simulink model "PathPlanning"  (R2025a)
settings: Solver=FixedStepAuto  StartTime=0.0  StopTime=10  FixedStep=1  RelTol=1e-3  EnableMultiTasking=on
undefined symbols (not defined in the file): costMap, finalPose, geometry, initialPose, metric, samplingBoxCenterPose, samplingBoxDimension, verticesStaticObstacles
libraries: MPSV x3
settings Model: Creator=damerius  LastModifiedBy=damerius
settings SolverCC: ConcurrentTasks=on  AlgebraicLoopSolver=TrustRegion  PositivePriorityOrder=on
settings DataIOCC: SaveOutput=off  SignalLogging=off  DSMLogging=off  SaveTime=off  ReturnWorkspaceOutputs=off
settings OptimizationCC: DefaultParameterBehavior=Inlined  ReuseModelBlockBuffer=off  ZeroExternalMemoryAtStartup=off  ZeroInternalMemoryAtStartup=off  SimCompilerOptimization=on
settings DebuggingCC: UnconnectedInputMsg=warning  UnconnectedOutputMsg=warning  UnconnectedLineMsg=warning
settings HardwareCC: ProdBitPerLong=64.0  ProdHWDeviceType=Intel->x86-64 (Linux 64)
settings ModelReferenceCC: EnableRefExpFcnMdlSchedulingChecks=on
settings SFSimCC: SimParseCustomCode=off  SimGenImportedTypeDefs=on  SimTargetLang=C++  SimDLTargetLibrary=mkl-dnn
settings RTWCC: GenCodeOnly=on  PackageGeneratedCodeAndArtifacts=on  PackageName=PackNGo  RTWVerbose=off  BuildConfiguration=Faster Runs  TargetLang=C++  GPUComputeCapability=3.5  DLArmComputeVersion=19.05
settings CodeAppCC: ForceParamTrailComments=on  MaxIdLength=95.0  MATLABSourceComments=on  UseSimReservedNames=on
settings GRTTargetCC: TargetLangStandard=C++11 (ISO)  GenerateFullHeader=off  MatFileLogging=off  CodeInterfacePackaging=C++ class  SubcomponentCodeInterfacePackaging=C++ class

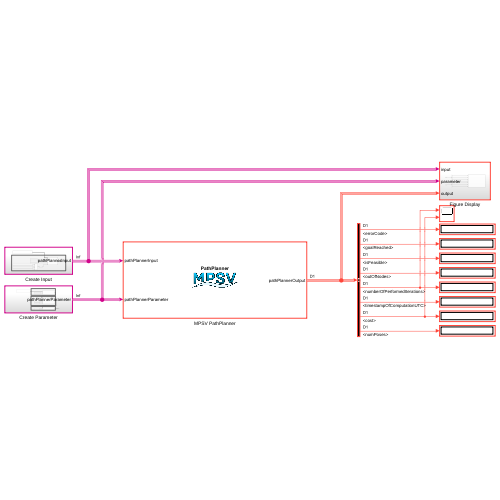
[thumbnail: Simulink's stored preview of the top-level diagram]
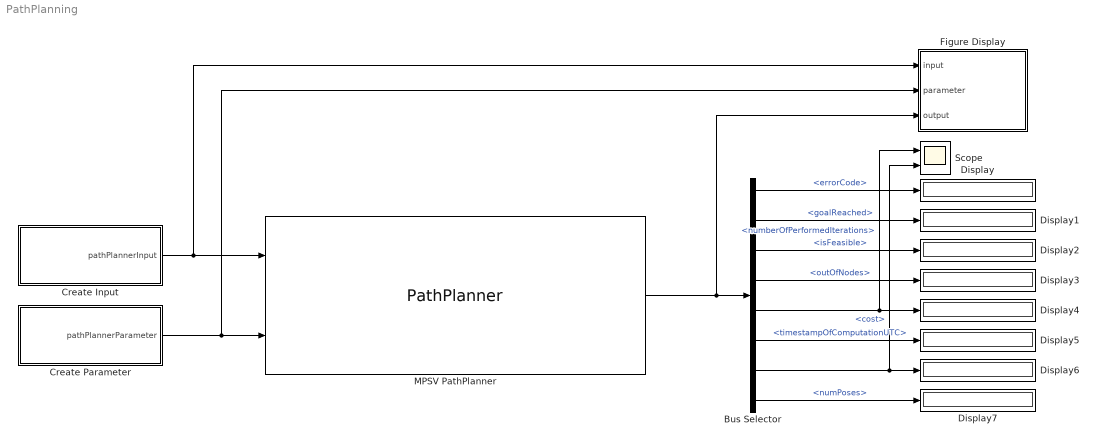
== system PathPlanning ==
  Bus Selector : BusSelector  OutputSignals=errorCode,goalReached,isFeasible,outOfNodes,numberOfPerformedIterations,timestampOfComputationUTC,cost,numPoses
  Create Input : Subsystem
  Create Parameter : Subsystem
  Display{,1..7} (8 alike) : Display
  Figure Display : Subsystem
  MPSV PathPlanner : MPSV/PathPlanner  maxNumNodes=1000  maxNumSamples=1000000
      settings: SourceProductName=MPSV - Motion Planner for Surface Vehicles
  Scope : Scope  NumInputPorts=2
      settings: ActiveDisplayYMinimum=19472  ActiveDisplayYMaximum=20852
  wires:
  MPSV PathPlanner/1 -> Figure Display/3(output), Bus Selector/1
  Bus Selector/8 -> Display7/1  "<numPoses>"
  Bus Selector/7 -> Scope/2, Display6/1  "<cost>"
  Bus Selector/6 -> Display5/1  "<timestampOfComputationUTC>"
  Bus Selector/5 -> Scope/1, Display4/1  "<numberOfPerformedIterations>"
  Create Input/1(pathPlannerInput) -> Figure Display/1(input), MPSV PathPlanner/1
  Create Parameter/1(pathPlannerParameter) -> Figure Display/2(parameter), MPSV PathPlanner/2
  Bus Selector/1 -> Display/1  "<errorCode>"
  Bus Selector/2 -> Display1/1  "<goalReached>"
  Bus Selector/3 -> Display2/1  "<isFeasible>"
  Bus Selector/4 -> Display3/1  "<outOfNodes>"

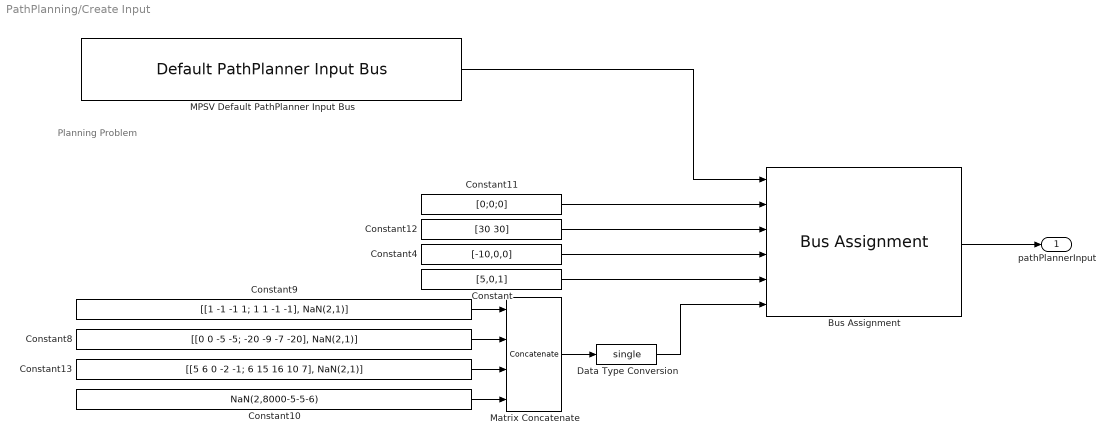
== system PathPlanning/Create Input ==
  note: Planning Problem
  Bus Assignment : BusAssignment  AssignedSignals=samplingBoxCenterPose,samplingBoxDimension,initialPose,finalPose,verticesStaticObstacles
  Constant : Constant  Value=[5,0,1]
  Constant10 : Constant  Value=NaN(2,8000-5-5-6)
  Constant11 : Constant  Value=[0;0;0]
  Constant12 : Constant  Value=[30 30]
  Constant13 : Constant  Value=[[5 6 0 -2 -1; 6 15 16 10 7], NaN(2,1)]
  Constant4 : Constant  Value=[-10,0,0]
  Constant8 : Constant  Value=[[0 0 -5 -5; -20 -9 -7 -20], NaN(2,1)]
  Constant9 : Constant  Value=[[1 -1 -1 1; 1 1 -1 -1], NaN(2,1)]
  Data Type Conversion : DataTypeConversion  OutDataTypeStr=single  SaturateOnIntegerOverflow=off  RndMeth=Floor
  MPSV Default PathPlanner Input Bus : MPSV/Default PathPlanner Input Bus
      settings: SourceProductName=MPSV - Motion Planner for Surface Vehicles
  Matrix Concatenate : Concatenate  NumInputs=4  Mode=Multidimensional array  ConcatenateDimension=2
  pathPlannerInput : Outport
  wires:
  Constant11/1 -> Bus Assignment/2
  Constant/1 -> Bus Assignment/5
  Constant4/1 -> Bus Assignment/4
  MPSV Default PathPlanner Input Bus/1 -> Bus Assignment/1
  Constant12/1 -> Bus Assignment/3
  Bus Assignment/1 -> pathPlannerInput/1
  Constant8/1 -> Matrix Concatenate/2
  Constant13/1 -> Matrix Concatenate/3
  Constant10/1 -> Matrix Concatenate/4
  Constant9/1 -> Matrix Concatenate/1
  Matrix Concatenate/1 -> Data Type Conversion/1
  Data Type Conversion/1 -> Bus Assignment/6

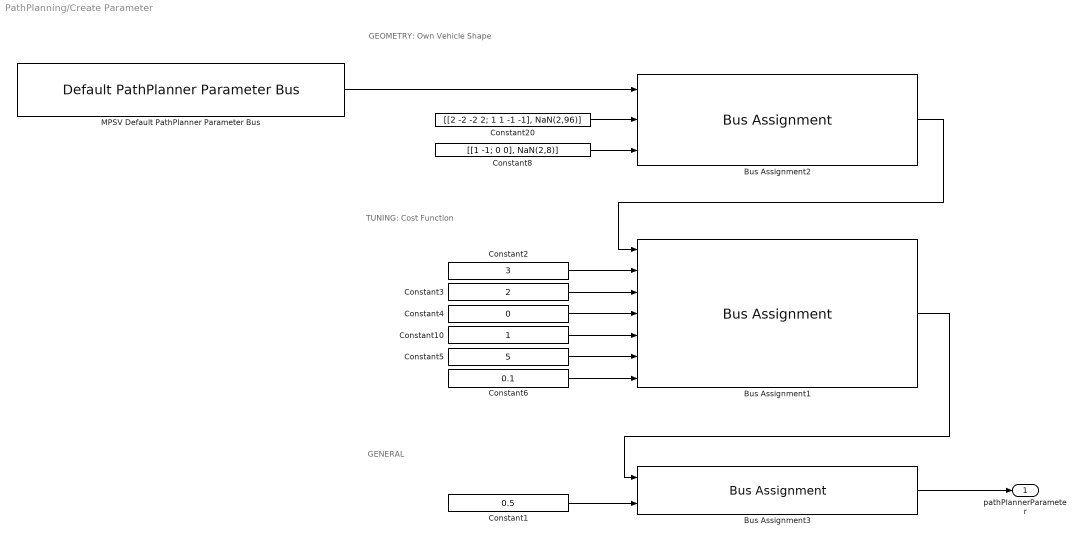
== system PathPlanning/Create Parameter ==
  note: GEOMETRY: Own Vehicle Shape
  note: TUNING: Cost Function
  note: GENERAL
  Bus Assignment1 : BusAssignment  AssignedSignals=metric.weightPsi,metric.weightSway,metric.weightReverseScale,metric.weightReverseDecay,costMap.distanceScale,costMap.distanceDecay
  Bus Assignment2 : BusAssignment  AssignedSignals=geometry.verticesVehicleShape,geometry.skeletalPoints
  Bus Assignment3 : BusAssignment  AssignedSignals=pathPlanner.maxComputationTime
  Constant1 : Constant  Value=0.5
  Constant10 : Constant
  Constant2 : Constant  Value=3
  Constant20 : Constant  Value=[[2 -2 -2 2; 1 1 -1 -1], NaN(2,96)]  OutDataTypeStr=single
  Constant3 : Constant  Value=2
  Constant4 : Constant  Value=0
  Constant5 : Constant  Value=5
  Constant6 : Constant  Value=0.1
  Constant8 : Constant  Value=[[1 -1; 0 0], NaN(2,8)]  OutDataTypeStr=single
  MPSV Default PathPlanner Parameter Bus : MPSV/Default PathPlanner Parameter Bus
      settings: SourceProductName=MPSV - Motion Planner for Surface Vehicles
  pathPlannerParameter : Outport
  wires:
  Constant8/1 -> Bus Assignment2/3
  Constant5/1 -> Bus Assignment1/6
  MPSV Default PathPlanner Parameter Bus/1 -> Bus Assignment2/1
  Constant1/1 -> Bus Assignment3/2
  Constant2/1 -> Bus Assignment1/2
  Bus Assignment1/1 -> Bus Assignment3/1
  Bus Assignment2/1 -> Bus Assignment1/1
  Constant6/1 -> Bus Assignment1/7
  Constant3/1 -> Bus Assignment1/3
  Bus Assignment3/1 -> pathPlannerParameter/1
  Constant4/1 -> Bus Assignment1/4
  Constant10/1 -> Bus Assignment1/5
  Constant20/1 -> Bus Assignment2/2

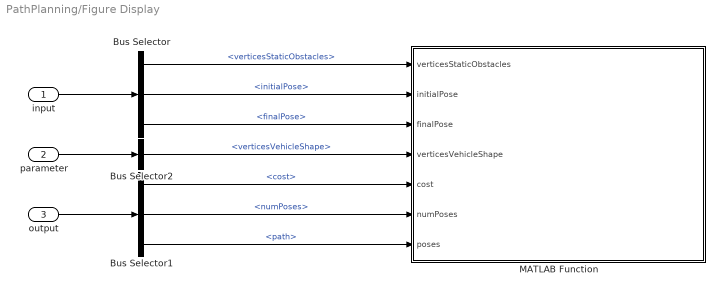
== system PathPlanning/Figure Display ==
  input : Inport
  parameter : Inport  Port=2
  output : Inport  Port=3
  Bus Selector : BusSelector  OutputSignals=verticesStaticObstacles,initialPose,finalPose
  Bus Selector1 : BusSelector  OutputSignals=cost,numPoses,path
  Bus Selector2 : BusSelector  OutputSignals=geometry.verticesVehicleShape
  MATLAB Function : MATLAB Function  TreatAsAtomicUnit=on
  wires:
  parameter/1 -> Bus Selector2/1
  input/1 -> Bus Selector/1
  Bus Selector/1 -> MATLAB Function/1(verticesStaticObstacles)  "<verticesStaticObstacles>"
  Bus Selector/2 -> MATLAB Function/2(initialPose)  "<initialPose>"
  Bus Selector/3 -> MATLAB Function/3(finalPose)  "<finalPose>"
  output/1 -> Bus Selector1/1
  Bus Selector1/1 -> MATLAB Function/5(cost)  "<cost>"
  Bus Selector1/2 -> MATLAB Function/6(numPoses)  "<numPoses>"
  Bus Selector1/3 -> MATLAB Function/7(poses)  "<path>"
  Bus Selector2/1 -> MATLAB Function/4(verticesVehicleShape)  "<verticesVehicleShape>"

== matlab function PathPlanning/Figure Display/MATLAB Function ==
  data: verticesStaticObstacles input; initialPose input; finalPose input; verticesVehicleShape input; cost input; numPoses input; poses input
function FigureDisplay(verticesStaticObstacles, initialPose, finalPose, verticesVehicleShape, cost, numPoses, poses)
    persistent f;
    if(isempty(f))
        f = figure(42);
    end

    clf;
    hold on;
    PlotPath(numPoses, poses, verticesVehicleShape, [0 0.3 0.5]);
    PlotVehicleShape(initialPose, verticesVehicleShape, [0.9 0 0]);
    PlotVehicleShape(finalPose, verticesVehicleShape, [0 0.7 0]);
    PlotObstacles(verticesStaticObstacles);
    view(90,-90);
    axis equal;
    box on;
    grid on;
    xlabel('x in m');
    ylabel('y in m');
    title(sprintf('cost: %f',cost));
    drawnow();
end

function PlotPath(numPoses, poses, verticesVehicleShape, color)
    x = poses(1,1:numPoses);
    y = poses(2,1:numPoses);
    plot(x,y,'LineWidth',2,'Color',color);
    for i = uint32(1):uint32(numPoses)
        PlotVehicleShape(poses(:,i), verticesVehicleShape, color);
    end
end

function PlotVehicleShape(pose, verticesVehicleShape, color)
    c = cos(pose(3));
    s = sin(pose(3));
    R = [c -s; s c];

    N = int32(size(verticesVehicleShape,2));
    i0 = int32(-1);

    for i = int32(1):N
        finiteVertex = isfinite(verticesVehicleShape(1,i)) && isfinite(verticesVehicleShape(2,i));
        if((i0 < 1) && finiteVertex)
            i0 = i;
        elseif((i0 > 0) && (~finiteVertex || (i == N)))
            i = i + int32((i == N) && finiteVertex);
            vertices = R * verticesVehicleShape(:,i0:(i-1)) + [pose(1); pose(2)];
            PlotPolygon(vertices, color);
            plot(pose(1),pose(2),'o','Color',color);
            i0 = int32(-1);
        end
    end
end

function PlotObstacles(verticesStaticObstacles)
    N = int32(size(verticesStaticObstacles,2));
    i0 = int32(-1);

    for i = int32(1):N
        finiteVertex = isfinite(verticesStaticObstacles(1,i)) && isfinite(verticesStaticObstacles(2,i));
        if((i0 < 1) && finiteVertex)
            i0 = i;
        elseif((i0 > 0) && (~finiteVertex || (i == N)))
            i = i + int32((i == N) && finiteVertex);
            PlotPolygon(verticesStaticObstacles(:,i0:(i-1)), [0,0,0]);
            i0 = int32(-1);
        end
    end
end

function PlotPolygon(vertices, color)
    x = [vertices(1,:) vertices(1,1)];
    y = [vertices(2,:) vertices(2,1)];
    plot(x,y,'LineWidth',1,'Color',color);
end
